simulink model "ACC_Duty"  (R2021b)
settings: Solver=FixedStepAuto  StartTime=0.0  StopTime=inf  FixedStep=0.01  RelTol=1e-3  EnableMultiTasking=on
libraries: arduinolib x5, simulink x2, arduinosensorlib x1
settings Model: ExtModeTrigDuration=2  Creator=user  LastModifiedBy=user
settings OptimizationCC: EnhancedBackFolding=on  PassReuseOutputArgsAs=Individual arguments  ZeroExternalMemoryAtStartup=off  ZeroInternalMemoryAtStartup=off  MaxStackSize=64  OptimizeBlockOrder=speed  DifferentSizesBufferReuse=on  OptimizationCustomize=off  EfficientTunableParamExpr=on
settings DebuggingCC: ParameterTunabilityLossMsg=error
settings HardwareCC: ProdBitPerInt=16  ProdBitPerPointer=16  ProdBitPerSizeT=16  ProdBitPerPtrDiffT=16  ProdLargestAtomicFloat=None  ProdWordSize=8  ProdHWDeviceType=Atmel->AVR
settings SFSimCC: MATLABDynamicMemAlloc=off
settings RTWCC: Description=Embedded Coder  SystemTargetFile=ert.tlc  HardwareBoard=Arduino Mega 2560  TemplateMakefile=ert_default_tmf  Toolchain=Arduino AVR  BuildConfiguration=Faster Runs
settings CodeAppCC: ForceParamTrailComments=on  IgnoreCustomStorageClasses=off  OperatorAnnotations=on  SimulinkDataObjDesc=on  SFDataObjDesc=on  InsertBlockDesc=on
settings ERTTargetCC: SupportContinuousTime=on  SupportVariableSizeSignals=on  ExtModeTransport=3  ExtModeStaticAlloc=on  ExtModeStaticAllocSize=2048  ExtModeMexFile=ext_xcp  ExtModeIntrfLevel=Level2 - Open

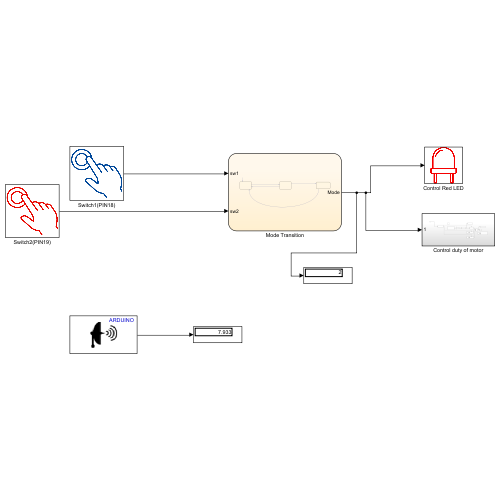
[thumbnail: Simulink's stored preview of the top-level diagram]
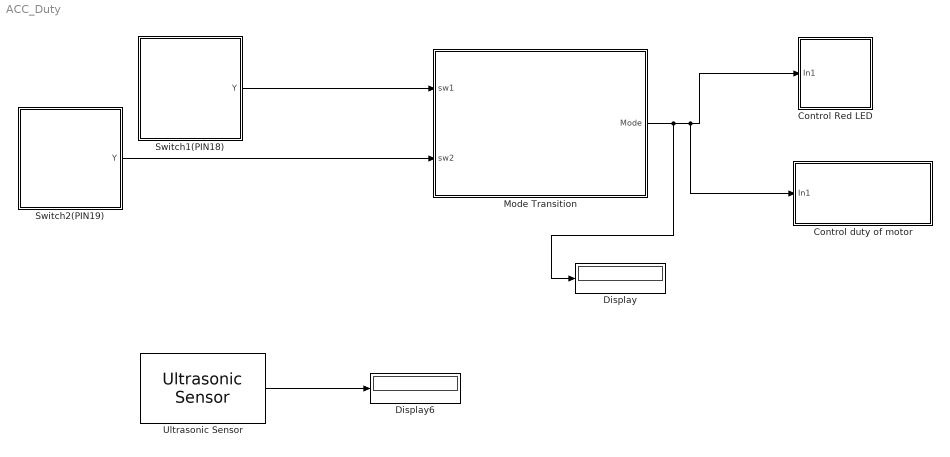
== system ACC_Duty ==
  Control Red LED : Subsystem
      mask Display: image('C:\Users\user\Downloads\led-bulb.png'); % 변경하려면 툴스트립에 있는 "이미지 편집"을 사용하십시오.
  Control duty of motor : Subsystem
  Display : Display
  Display6 : Display
  Mode Transition : Stateflow chart  TreatAsAtomicUnit=on
  Switch1(PIN18) : Subsystem
      mask Display: image('C:\Users\user\Downloads\button (2).png'); % 변경하려면 툴스트립에 있는 "이미지 편집"을 사용하십시오.
  Switch2(PIN19) : Subsystem
      mask Display: image('C:\Users\user\Downloads\button (3).png'); % 변경하려면 툴스트립에 있는 "이미지 편집"을 사용하십시오.
  Ultrasonic Sensor : arduinosensorlib/Ultrasonic Sensor  NumSignalPins=2  TrigPin=50  EchoPin=51  SignalPin=3  SampleTime_=0.1  blockPlatform=ARDUINO
      settings: SourceProductBaseCode=ARDUINO
  wires:
  Mode Transition/1(Mode) -> Display/1, Control duty of motor/1(In1), Control Red LED/1(In1)
  Ultrasonic Sensor/1 -> Display6/1
  Switch1(PIN18)/1(Y) -> Mode Transition/1(sw1)
  Switch2(PIN19)/1(Y) -> Mode Transition/2(sw2)

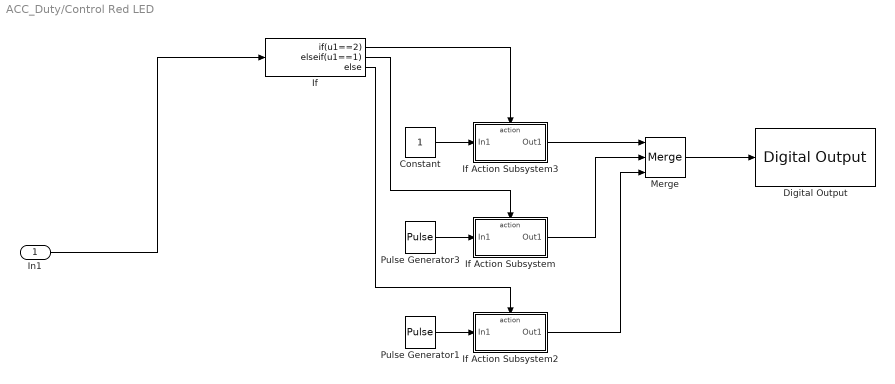
== system ACC_Duty/Control Red LED ==
  In1 : Inport
  Constant : Constant
  Digital Output : arduinolib/Digital Output  pinNumber=12  Direction=output  blockPlatform=arduino
  If : If  IfExpression=u1==2  ElseIfExpressions=u1==1
  If Action Subsystem : Subsystem  TreatAsAtomicUnit=on
  If Action Subsystem2 : Subsystem  TreatAsAtomicUnit=on
  If Action Subsystem3 : Subsystem  TreatAsAtomicUnit=on
  Merge : Merge  Inputs=3
  Pulse Generator1 : DiscretePulseGenerator  Period=20  PulseWidth=10  SampleTime=-1
  Pulse Generator3 : DiscretePulseGenerator  Period=4  PulseWidth=2  SampleTime=-1
  wires:
  If Action Subsystem2/1(Out1) -> Merge/3
  Pulse Generator1/1 -> If Action Subsystem2/1(In1)
  Pulse Generator3/1 -> If Action Subsystem/1(In1)
  Merge/1 -> Digital Output/1
  If Action Subsystem/1(Out1) -> Merge/2
  If/1 -> If Action Subsystem3/Action
  If/2 -> If Action Subsystem/Action
  Constant/1 -> If Action Subsystem3/1(In1)
  If/3 -> If Action Subsystem2/Action
  If Action Subsystem3/1(Out1) -> Merge/1
  In1/1 -> If/1

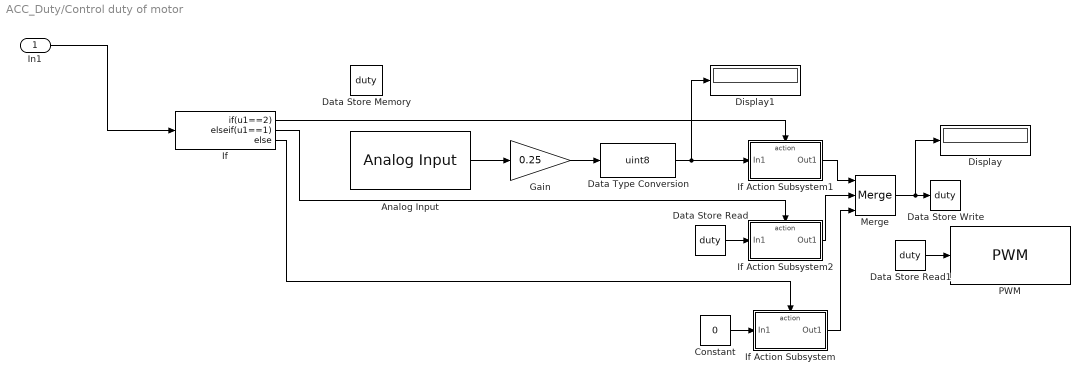
== system ACC_Duty/Control duty of motor ==
  In1 : Inport
  Analog Input : arduinolib/Analog Input  pinNumber=0  ReadResultsOnly=off  ConversionTriggerSource=Software  ExternalTriggerType=uint32( 0 )  OutputDataType=uint16  EnableConversionCompleteNotify=off  EnableOuputStatus=off  SampleTime=-1  blockPlatform=arduino
  Constant : Constant  Value=0  OutDataTypeStr=uint8
  Data Store Memory : DataStoreMemory  DataStoreName=duty  ReadBeforeWriteMsg=warning  WriteAfterWriteMsg=warning  WriteAfterReadMsg=warning  ShowAdditionalParam=off  OutDataTypeStr=uint8
  Data Store Read : DataStoreRead  DataStoreName=duty  IndexOptions=Index vector (dialog)  Indices=1  OutputSizes=1
  Data Store Read1 : DataStoreRead  DataStoreName=duty  IndexOptions=Index vector (dialog)  Indices=1  OutputSizes=1
  Data Store Write : DataStoreWrite  DataStoreName=duty  IndexOptions=Index vector (dialog)  Indices=1  OutputSizes=1
  Data Type Conversion : DataTypeConversion  OutDataTypeStr=uint8
  Display : Display
  Display1 : Display
  Gain : Gain  Gain=0.25
  If : If  IfExpression=u1==2  ElseIfExpressions=u1==1
  If Action Subsystem : Subsystem  TreatAsAtomicUnit=on
  If Action Subsystem1 : Subsystem  TreatAsAtomicUnit=on
  If Action Subsystem2 : Subsystem  TreatAsAtomicUnit=on
  Merge : Merge  Inputs=3
  PWM : arduinolib/PWM  pinNumber=11  frequencyType=Default  desiredFrequency=490.2  achievableFrequency=490.2
  wires:
  Data Type Conversion/1 -> If Action Subsystem1/1(In1), Display1/1
  Constant/1 -> If Action Subsystem/1(In1)
  If Action Subsystem2/1(Out1) -> Merge/2
  Gain/1 -> Data Type Conversion/1
  If/2 -> If Action Subsystem2/Action
  Analog Input/1 -> Gain/1
  Data Store Read1/1 -> PWM/1
  If/1 -> If Action Subsystem1/Action
  If/3 -> If Action Subsystem/Action
  If Action Subsystem1/1(Out1) -> Merge/1
  Data Store Read/1 -> If Action Subsystem2/1(In1)
  If Action Subsystem/1(Out1) -> Merge/3
  Merge/1 -> Display/1, Data Store Write/1
  In1/1 -> If/1

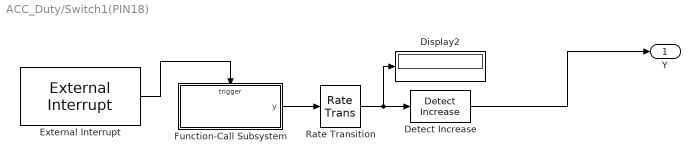
== system ACC_Duty/Switch1(PIN18) ==
  Detect Increase : simulink/Logic and Bit Operations/Detect Increase  vinit=0.0  OutDataTypeStr=boolean
  Display2 : Display
  External Interrupt : arduinolib/External Interrupt  Pin=18  PullUp=on  Mode=FALLING  InterruptSimulationInput=off
      settings: SourceProductBaseCode=ARDUINO
  Function-Call Subsystem : Subsystem  TreatAsAtomicUnit=on
  Rate Transition : RateTransition  Integrity=off  Deterministic=off
  Y : Outport
  wires:
  Function-Call Subsystem/1(y) -> Rate Transition/1
  Rate Transition/1 -> Display2/1, Detect Increase/1
  External Interrupt/1 -> Function-Call Subsystem/Trigger
  Detect Increase/1 -> Y/1

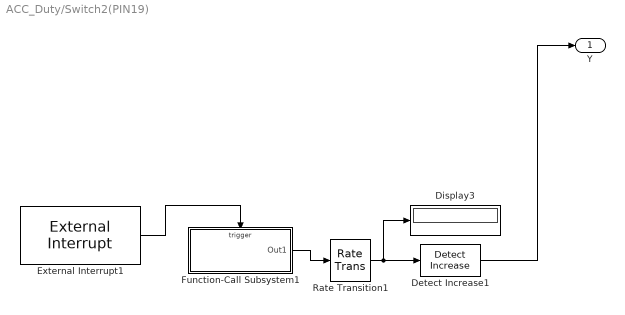
== system ACC_Duty/Switch2(PIN19) ==
  Detect Increase1 : simulink/Logic and Bit Operations/Detect Increase  vinit=0.0  OutDataTypeStr=uint8
  Display3 : Display
  External Interrupt1 : arduinolib/External Interrupt  Pin=19  PullUp=on  Mode=FALLING  InterruptSimulationInput=off
      settings: SourceProductBaseCode=ARDUINO
  Function-Call Subsystem1 : Subsystem  TreatAsAtomicUnit=on
  Rate Transition1 : RateTransition  Deterministic=off
  Y : Outport
  wires:
  Function-Call Subsystem1/1(Out1) -> Rate Transition1/1
  Rate Transition1/1 -> Display3/1, Detect Increase1/1
  External Interrupt1/1 -> Function-Call Subsystem1/Trigger
  Detect Increase1/1 -> Y/1

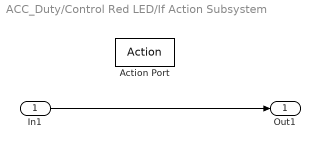
== system ACC_Duty/Control Red LED/If Action Subsystem ==
  In1 : Inport
  Action Port : ActionPort  ActionPortLabel=elseif(u1==1)
  Out1 : Outport
  wires:
  In1/1 -> Out1/1

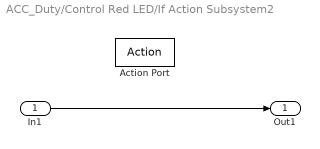
== system ACC_Duty/Control Red LED/If Action Subsystem2 ==
  In1 : Inport
  Action Port : ActionPort  ActionPortLabel=else
  Out1 : Outport
  wires:
  In1/1 -> Out1/1

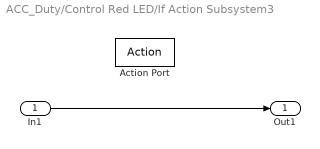
== system ACC_Duty/Control Red LED/If Action Subsystem3 ==
  In1 : Inport
  Action Port : ActionPort  ActionPortLabel=if(u1==2)
  Out1 : Outport
  wires:
  In1/1 -> Out1/1

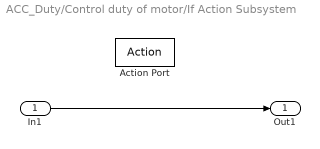
== system ACC_Duty/Control duty of motor/If Action Subsystem ==
  In1 : Inport
  Action Port : ActionPort  ActionPortLabel=else
  Out1 : Outport
  wires:
  In1/1 -> Out1/1

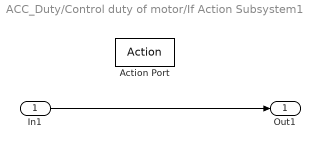
== system ACC_Duty/Control duty of motor/If Action Subsystem1 ==
  In1 : Inport
  Action Port : ActionPort  ActionPortLabel=if(u1==2)
  Out1 : Outport
  wires:
  In1/1 -> Out1/1

== system ACC_Duty/Control duty of motor/If Action Subsystem2 ==
  In1 : Inport
  Action Port : ActionPort  ActionPortLabel=elseif(u1==1)
  Out1 : Outport
  wires:
  In1/1 -> Out1/1

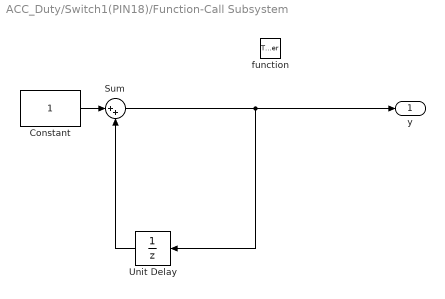
== system ACC_Duty/Switch1(PIN18)/Function-Call Subsystem ==
  function : TriggerPort  TriggerType=function-call  VariantControl=(inherit)
  Constant : Constant
  Sum : Sum  Inputs=|++
  Unit Delay : UnitDelay  SampleTime=-1  HasFrameUpgradeWarning=on
  y : Outport
  wires:
  Unit Delay/1 -> Sum/2
  Constant/1 -> Sum/1
  Sum/1 -> Unit Delay/1, y/1

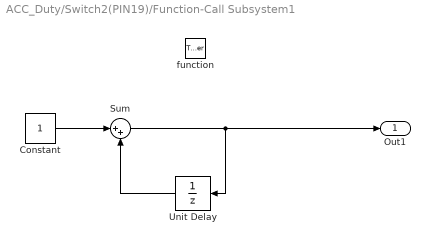
== system ACC_Duty/Switch2(PIN19)/Function-Call Subsystem1 ==
  function : TriggerPort  TriggerType=function-call  VariantControl=(inherit)
  Constant : Constant
  Sum : Sum  Inputs=|++
  Unit Delay : UnitDelay  SampleTime=-1  HasFrameUpgradeWarning=on
  Out1 : Outport
  wires:
  Sum/1 -> Unit Delay/1, Out1/1
  Unit Delay/1 -> Sum/2
  Constant/1 -> Sum/1

== stateflow chart ACC_Duty/Mode Transition ==
  state ACC_off
    Mode=0;
  state ACC_standby
    Mode=1;
  state ACC_active
    Mode=2;
  (default) -> ACC_off
  ACC_standby -> ACC_active [order 2] : [sw1==1 ]
  ACC_off -> ACC_standby : [sw1==1 ]
  ACC_standby -> ACC_off [order 1] : [sw2==1]
  ACC_active -> ACC_off : [sw1 == 1 || sw2 ==1]
  data: Mode output; sw1 input; sw2 input
